simulink model "Robot_control"  (R2020b)
settings: Solver=FixedStepAuto  StartTime=0.0  StopTime=inf  FixedStep=0.01  RelTol=1e-3
values from neighbouring files (symbols this model uses):
  Initial_pos = [20 20 10]    [Robot_control_script.m]
  min_pwm_change = 0.39    [Robot_control_script.m]
  Motorspeed_MG996 = 60/.17    (= 352.941176471)    [Robot_control_script.m]
  Time_to_wait = [1 10]    [Robot_control_script.m]
  weights = [1 1 1 1 1 1]    [Robot_control_script.m]
undefined symbols (not defined in the file or in its folder): DiscIntNeverNeededParam, Levenberg, Marquardt, read_the_data, send_serial, Serial_Port, Standard_Devices
libraries: sldrtlib x4, simulink x3, robotcorelib x2, robotmaniplib x1, simulink_extras x1, dspstat3 x1, mspfiltlib x1, dspfdesign x1
(part 1 of 2)
settings Model: Creator=jsmit  LastModifiedBy=jsmit
settings OptimizationCC: DefaultParameterBehavior=Inlined  UseDivisionForNetSlopeComputation=on  GainParamInheritBuiltInType=on  UseFloatMulNetSlope=on  InlineInvariantSignals=on  EnhancedBackFolding=on  PassReuseOutputArgsAs=Individual arguments  ZeroExternalMemoryAtStartup=off  ZeroInternalMemoryAtStartup=off  EfficientFloat2IntCast=on  OptimizeBlockOrder=speed  DifferentSizesBufferReuse=on  OptimizationCustomize=off  EfficientTunableParamExpr=on
settings DebuggingCC: ParameterTunabilityLossMsg=error
settings SFSimCC: MATLABDynamicMemAllocThreshold=400000
settings RTWCC: Description=Embedded Coder  SystemTargetFile=ert.tlc  GenerateMakefile=off  TemplateMakefile=ert_default_tmf  GenerateReport=on  LaunchReport=on  TargetLang=C++  RTWCompilerOptimization=on
settings CodeAppCC: ForceParamTrailComments=on  IgnoreCustomStorageClasses=off  MaxIdLength=95  OperatorAnnotations=on  SimulinkDataObjDesc=on  SFDataObjDesc=on  InsertBlockDesc=on
settings ERTTargetCC: TargetLangStandard=C++03 (ISO)  GenerateSampleERTMain=on  CodeInterfacePackaging=C++ class  InlinedParameterPlacement=NonHierarchical  RootIOFormat=Structure reference  ERTCustomFileTemplate=example_file_process.tlc

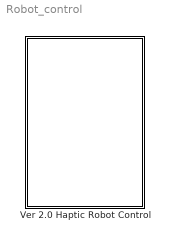
== system Robot_control ==
  Ver 2.0 Haptic Robot Control : Subsystem

== system Robot_control/Ver 2.0 Haptic Robot Control ==
  Motor Driver System : Subsystem
  Tooltip System : Subsystem  Commented=on

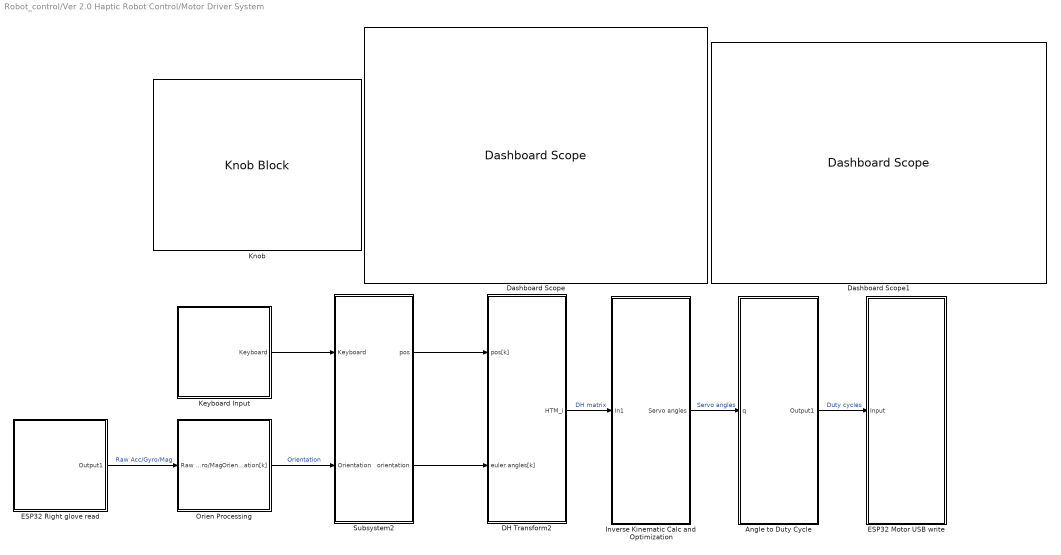
== system Robot_control/Ver 2.0 Haptic Robot Control/Motor Driver System ==
  Angle to Duty Cycle : Subsystem
  DH Transform2 : Subsystem
  Dashboard Scope : DashboardScope  TimeSpan=60  Ymin=-50  Ymax=50
  Dashboard Scope1 : DashboardScope  TimeSpan=60  Ymin=-180  Ymax=180
  ESP32 Motor USB write : Subsystem
  ESP32 Right glove read : Subsystem
  Inverse Kinematic Calc and Optimization : Subsystem
  Keyboard Input : Subsystem
  Knob : KnobBlock  ScaleMin=-40  ScaleMax=40
  Orien Processing : Subsystem
  Subsystem2 : Subsystem
  wires:
  Inverse Kinematic Calc and Optimization/1(Servo angles) -> Angle to Duty Cycle/1(q)  "Servo angles"
  Angle to Duty Cycle/1(Output1) -> ESP32 Motor USB write/1(Input)  "Duty cycles"
  ESP32 Right glove read/1(Output1) -> Orien Processing/1(Raw Acc/Gyro/Mag)  "Raw Acc/Gyro/Mag"
  DH Transform2/1(HTM_i) -> Inverse Kinematic Calc and Optimization/1(In1)  "DH matrix"
  Keyboard Input/1(Keyboard) -> Subsystem2/1(Keyboard)
  Orien Processing/1(Orientation[k]) -> Subsystem2/2(Orientation)  "Orientation"
  Subsystem2/1(pos) -> DH Transform2/1(pos[k])
  Subsystem2/2(orientation) -> DH Transform2/2(euler angles[k])

== system Robot_control/Ver 2.0 Haptic Robot Control/Tooltip System ==
  Constant : Constant  Value=100
  Counter Limited : simulink/Sources/Counter Limited  uplimit=100  tsamp=-1
  Display : Display
  ESP32 Motor USB write : Subsystem  Commented=on
  ESP32 Tooltip USB read : Subsystem
  GreaterThan : RelationalOperator  Operator===  OutDataTypeStr=boolean  RndMeth=Simplest
  Laser and Touch Processing : Subsystem  Commented=on
  Subsystem : Subsystem
  Subsystem1 : Subsystem
  wires:
  Laser and Touch Processing/1(Laser distance filtered/touch) -> ESP32 Motor USB write/1(Input)  "Tooltip Data"
  ESP32 Tooltip USB read/1(Distance/Touch) -> Subsystem1/1(Tooltip data), Laser and Touch Processing/1(Input)  "Tooltip data"
  GreaterThan/1 -> Display/1, Subsystem/Enable
  Counter Limited/1 -> GreaterThan/1
  Constant/1 -> GreaterThan/2
  Subsystem1/1(y) -> Subsystem/1(Input)

== system Robot_control/Ver 2.0 Haptic Robot Control/Motor Driver System/Angle to Duty Cycle ==
  q : Inport
  Add : Sum
  Constant : Constant  Value=0.025/60
  Constant1 : Constant  Value=0.075
  Display : Display
  Display1 : Display
  Product : Product
  Output1 : Outport
  wires:
  q/1 -> Product/2  "q"
  Constant/1 -> Product/1
  Product/1 -> Display/1, Add/2
  Constant1/1 -> Add/1
  Add/1 -> Display1/1, Output1/1  "Duty Cycle"

== system Robot_control/Ver 2.0 Haptic Robot Control/Motor Driver System/DH Transform2 ==
  pos[k] : Inport
  euler angles[k] : Inport  Port=2
  Coordinate Transformation Conversion : robotcorelib/Coordinate Transformation Conversion  InputRepresentation=Euler Angles  InputEulerSequence=XYZ  ShowTrVecInputPort=on  OutputRepresentation=Homogeneous Transformation  OutputEulerSequence=ZYX  ShowTrVecOutputPort=on  SimulateUsing=Interpreted execution
      settings: SourceProductBaseCode=NV,RO,RR,UV
  HTM_i : Outport
  wires:
  Coordinate Transformation Conversion/1 -> HTM_i/1  "i-1_A_i"
  euler angles[k]/1 -> Coordinate Transformation Conversion/1  "Euler Angles[k]"
  pos[k]/1 -> Coordinate Transformation Conversion/2  "Pos[k]"

== system Robot_control/Ver 2.0 Haptic Robot Control/Motor Driver System/ESP32 Motor USB write ==
  Input : Inport  PortDimensions=6
  Constant : Constant  Value=100
  Counter Limited : simulink/Sources/Counter Limited  uplimit=100  tsamp=-1
  Display : Display
  GreaterThan : RelationalOperator  Operator===  OutDataTypeStr=boolean  RndMeth=Simplest
  Subsystem : Subsystem
  wires:
  Constant/1 -> GreaterThan/2
  Counter Limited/1 -> GreaterThan/1
  Input/1 -> Subsystem/1(Input)  "PWM values"
  GreaterThan/1 -> Display/1, Subsystem/Enable

== system Robot_control/Ver 2.0 Haptic Robot Control/Motor Driver System/ESP32 Right glove read ==
  Triggered Subsystem : Subsystem  TreatAsAtomicUnit=on
  Output1 : Outport
  wires:
  Triggered Subsystem/1(y) -> Output1/1  "Glove Data"

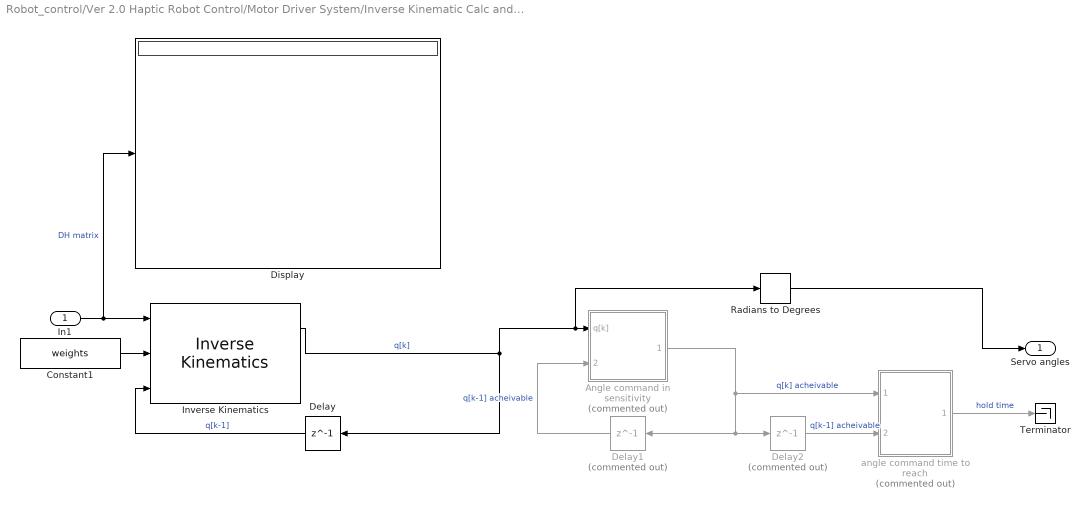
== system Robot_control/Ver 2.0 Haptic Robot Control/Motor Driver System/Inverse Kinematic Calc and Optimization ==
  In1 : Inport
  Angle command in sensitivity : Subsystem  Commented=on
  Constant1 : Constant  Value=weights
  Delay : Delay  DelayLength=1
  Delay1 : Delay  Commented=on  DelayLength=1
  Delay2 : Delay  Commented=on  DelayLength=1
  Display : Display
  Inverse Kinematics : robotmaniplib/Inverse Kinematics  RigidBodyTree=robot  EndEffector=body6  ShowInfo=off  SolverName=Levenberg-Marquardt  EnforceJointLimits=on  MaxIterations=10  MaxTime=0.3  GradientTolerance=1e-7  SolutionTolerance=0.1  StepTolerance=1e-14  ErrorChangeTolerance=0.1  UseErrorDamping=on  DampingBias=0.0025  SimulateUsing=Interpreted execution
  Radians to Degrees : simulink_extras/Transformations/Radians to Degrees
  Terminator : Terminator
  angle command time to reach : Subsystem  Commented=on
  Servo angles : Outport
  wires:
  Constant1/1 -> Inverse Kinematics/2
  Inverse Kinematics/1 -> Radians to Degrees/1, Angle command in sensitivity/1(q[k]), Delay/1  "q[k]"
  In1/1 -> Display/1, Inverse Kinematics/1  "DH matrix"
  Delay/1 -> Inverse Kinematics/3  "q[k-1]"
  Angle command in sensitivity/1(q[k] acheivable) -> Delay2/1, Delay1/1, angle command time to reach/1(q[k] acheivable)  "q[k] acheivable"
  Delay1/1 -> Angle command in sensitivity/2(q[k-1] acheivable)  "q[k-1] acheivable"
  Delay2/1 -> angle command time to reach/2(q[k-1] acheivable)  "q[k-1] acheivable"
  angle command time to reach/1(Output) -> Terminator/1  "hold time"
  Radians to Degrees/1 -> Servo angles/1

== system Robot_control/Ver 2.0 Haptic Robot Control/Motor Driver System/Keyboard Input ==
  Keyboard 1 : M-S-Function  FunctionName=sfun_keyboard_input_v1_2b  mask(Keyboard Input){}
      mask help: Keyboard Input
      mask Display: fprintf('Keyboard');
  Terminator : Terminator
  Keyboard : Outport
  wires:
  Keyboard 1/2 -> Terminator/1
  Keyboard 1/1 -> Keyboard/1

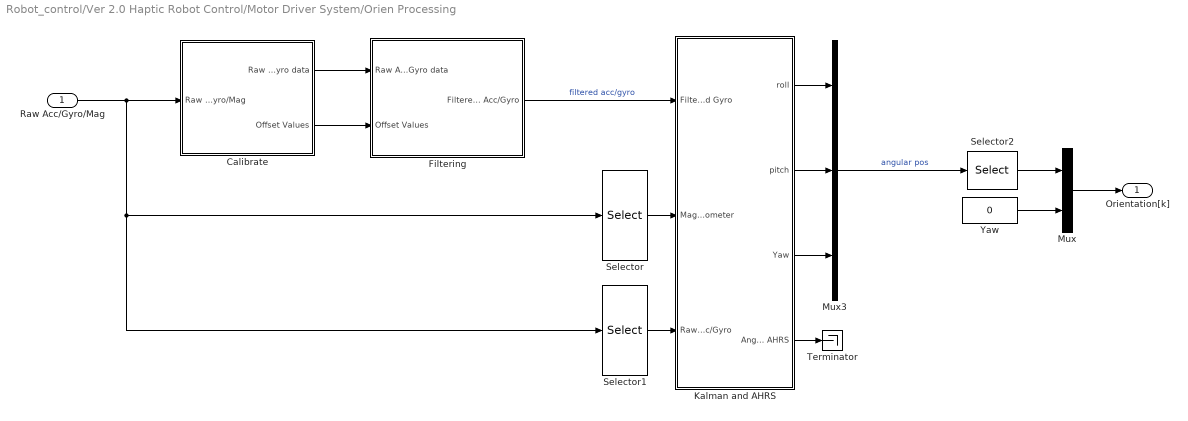
== system Robot_control/Ver 2.0 Haptic Robot Control/Motor Driver System/Orien Processing ==
  Raw Acc/Gyro/Mag : Inport
  Calibrate : Subsystem
  Filtering : Subsystem
  Kalman and AHRS : Subsystem
  Mux : Mux  Inputs=2
  Mux3 : Mux  Inputs=3
  Selector : Selector  InputPortWidth=9  IndexOptions=Index vector (dialog)  Indices=[7 8 9]  OutputSizes=1
  Selector1 : Selector  InputPortWidth=9  IndexOptions=Index vector (dialog)  Indices=[1 2 3 4 5 6]  OutputSizes=1
  Selector2 : Selector  InputPortWidth=3  IndexOptions=Index vector (dialog)  Indices=[1 2]  OutputSizes=1
  Terminator : Terminator
  Yaw : Constant  Value=0
  Orientation[k] : Outport
  wires:
  Filtering/1(Filtered Acc/Gyro) -> Kalman and AHRS/1(Filtered Acc and Gyro)  "filtered acc/gyro"
  Kalman and AHRS/3(Yaw) -> Mux3/3
  Kalman and AHRS/1(roll) -> Mux3/1
  Kalman and AHRS/2(pitch) -> Mux3/2
  Calibrate/1(Raw Acc/Gyro data) -> Filtering/1(Raw Acc/Gyro data)
  Raw Acc/Gyro/Mag/1 -> Selector1/1, Selector/1, Calibrate/1(Raw Acc/Gyro/Mag)
  Calibrate/2(Offset Values) -> Filtering/2(Offset Values)
  Mux3/1 -> Selector2/1  "angular pos"
  Selector/1 -> Kalman and AHRS/2(Magnetometer)
  Selector1/1 -> Kalman and AHRS/3(Raw Acc/Gyro)
  Selector2/1 -> Mux/1
  Mux/1 -> Orientation[k]/1
  Yaw/1 -> Mux/2
  Kalman and AHRS/4(Angular Velocity AHRS) -> Terminator/1

== system Robot_control/Ver 2.0 Haptic Robot Control/Motor Driver System/Subsystem2 ==
  Keyboard : Inport
  Orientation : Inport  Port=2
  NOT : Logic  Operator=NOT  IconShape=distinctive  AllPortsSameDT=off  OutDataTypeStr=boolean
  Saturation : Saturate  UpperLimit=40  LowerLimit=-40
  Select pos or orientation mode : Subsystem
  Subsystem : Subsystem
  pos : Outport
  orientation : Outport  Port=2
  wires:
  Select pos or orientation mode/2(pos) -> Saturation/1
  Orientation/1 -> Select pos or orientation mode/3(xy orientation), Subsystem/2(angular pos)
  NOT/1 -> Subsystem/Enable
  [A] -> Select pos or orientation mode/2(Keyboard)
  Select pos or orientation mode/3(orientation) -> orientation/1
  Select pos or orientation mode/1(In orientation mode) -> NOT/1
  Subsystem/1(xyz pos) -> Select pos or orientation mode/1(xy pos)
  [A] -> Subsystem/1(Keyboard)
  Keyboard/1 -> [A]
  Saturation/1 -> pos/1

== system Robot_control/Ver 2.0 Haptic Robot Control/Tooltip System/ESP32 Motor USB write ==
  Input : Inport  PortDimensions=6
  Constant : Constant  Value=100
  Counter Limited : simulink/Sources/Counter Limited  uplimit=100  tsamp=-1
  Display : Display
  GreaterThan : RelationalOperator  Operator===  OutDataTypeStr=boolean  RndMeth=Simplest
  Subsystem : Subsystem
  wires:
  Constant/1 -> GreaterThan/2
  Counter Limited/1 -> GreaterThan/1
  Input/1 -> Subsystem/1(Input)  "PWM values"
  GreaterThan/1 -> Display/1, Subsystem/Enable

== system Robot_control/Ver 2.0 Haptic Robot Control/Tooltip System/ESP32 Tooltip USB read ==
  Subsystem : Subsystem
  Distance/Touch : Outport
  wires:
  Subsystem/1(tool_data) -> Distance/Touch/1  "laser distance, touch"

== system Robot_control/Ver 2.0 Haptic Robot Control/Tooltip System/Laser and Touch Processing ==
  Input : Inport
  Demux : Demux  Outputs=2
  Lowpass Filter : dspfdesign/Lowpass Filter  FilterType=FIR  DesignForMinimumOrder=on  FilterOrder=50  PassbandFrequency=8e3  StopbandFrequency=12e3  PassbandRipple=0.1  StopbandAttenuation=80  InheritSampleRate=off  SampleRate=44100  SimulateUsing=Interpreted execution  roundingMode=Floor  coeffsDataTypeStr=fixdt(1,16)
  Mux : Mux  Inputs=2
  Subsystem : Subsystem
  Laser distance filtered/touch : Outport
  wires:
  Input/1 -> Demux/1  "Tooltip data[k]"
  Demux/1 -> Lowpass Filter/1  "Laser distance[k]"
  Lowpass Filter/1 -> Mux/1
  Mux/1 -> Laser distance filtered/touch/1
  Demux/2 -> Subsystem/1(Tiptouch[k])  "Tiptouch[k]"
  Subsystem/1(Tool touching last 3 samples) -> Mux/2

== system Robot_control/Ver 2.0 Haptic Robot Control/Tooltip System/Subsystem ==
  Input : Inport  PortDimensions=[1 2]
  Enable : EnablePort
  Display : Display
  Display1 : Display
  Interpreted MATLAB Function : MATLABFcn  MATLABFcn=send_serial(u)  OutputDimensions=0
  Stream Output1 : sldrtlib/Stream Output  Commented=on  SampleTime=0.01  MaxMissedTicks=inf  ShowMissedTicks=off  YieldWhenWaiting=off  DrvName=Standard_Devices/Serial_Port  DrvAddress=4  DrvOptions=[115200 8 0 0 0 0 0 0]  PortSizes=1  FormatString='%s'  ShowReady=off  ShowError=off  InitialValue=[]  FinalValue=[]
      settings: AttributesFormatString=Serial Port [4]  SourceProductBaseCode=WT
  wires:
  Input/1 -> Display1/1, Interpreted MATLAB Function/1

== system Robot_control/Ver 2.0 Haptic Robot Control/Tooltip System/Subsystem1 ==
  Tooltip data : Inport
  Display : Display
  Display1 : Display
  MATLAB Function1 : MATLAB Function  TreatAsAtomicUnit=on
  y : Outport  PortDimensions=[1 2]
  wires:
  Tooltip data/1 -> Display/1, MATLAB Function1/1(my_string)
  MATLAB Function1/1(y) -> Display1/1, y/1

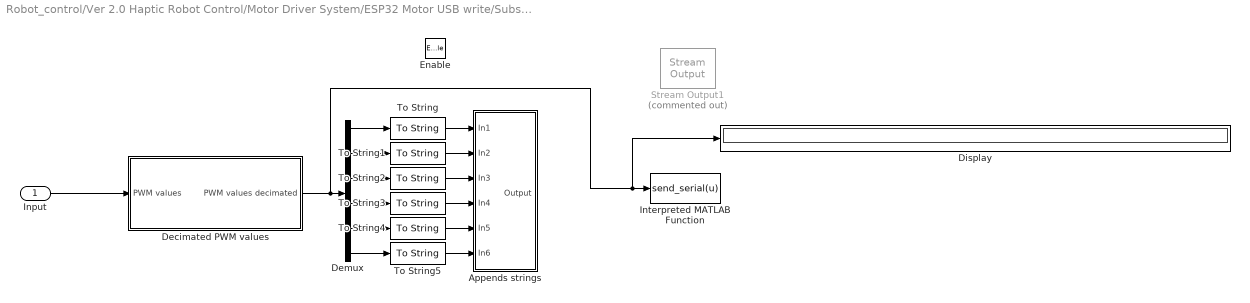
== system Robot_control/Ver 2.0 Haptic Robot Control/Motor Driver System/ESP32 Motor USB write/Subsystem ==
  Input : Inport  PortDimensions=6
  Enable : EnablePort
  Appends strings : Subsystem
  Decimated PWM values : Subsystem
  Demux : Demux  Outputs=6
  Display : Display
  Interpreted MATLAB Function : MATLABFcn  MATLABFcn=send_serial(u)  OutputDimensions=0
  Stream Output1 : sldrtlib/Stream Output  Commented=on  SampleTime=0.01  MaxMissedTicks=inf  ShowMissedTicks=off  YieldWhenWaiting=off  DrvName=Standard_Devices/Serial_Port  DrvAddress=4  DrvOptions=[115200 8 0 0 0 0 0 0]  PortSizes=1  FormatString='%s'  ShowReady=off  ShowError=off  InitialValue=[]  FinalValue=[]
      settings: AttributesFormatString=Serial Port [4]  SourceProductBaseCode=WT
  To String{,1..5} (6 alike) : ToString
  wires:
  Demux/3 -> To String2/1
  To String4/1 -> Appends strings/5(In5)
  Demux/6 -> To String5/1
  To String3/1 -> Appends strings/4(In4)
  Demux/1 -> To String/1
  To String2/1 -> Appends strings/3(In3)
  To String5/1 -> Appends strings/6(In6)
  To String1/1 -> Appends strings/2(In2)
  To String/1 -> Appends strings/1(In1)
  Demux/4 -> To String3/1
  Decimated PWM values/1(PWM values decimated) -> Display/1, Interpreted MATLAB Function/1, Demux/1
  Demux/2 -> To String1/1
  Demux/5 -> To String4/1
  Input/1 -> Decimated PWM values/1(PWM values)

== system Robot_control/Ver 2.0 Haptic Robot Control/Motor Driver System/ESP32 Right glove read/Triggered Subsystem ==
  Gain : Gain  Gain=1/100
  Interpreted MATLAB Function : MATLABFcn  Commented=on  MATLABFcn=read_the_data(u)
  MATLAB Function1 : MATLAB Function  TreatAsAtomicUnit=on
  Stream Input : sldrtlib/Stream Input  SampleTime=0.01  MaxMissedTicks=inf  ShowMissedTicks=off  YieldWhenWaiting=off  DrvName=Standard_Devices/Serial_Port  DrvAddress=8  DrvOptions=[9600 8 0 0 0 0 0 0]  DataTypes='string'  FormatString='%s'  Terminator={'\r', '\n'}  ShowReady=off  ShowError=off
      settings: AttributesFormatString=Serial Port [8]  SourceProductBaseCode=WT
  y : Outport  OutDataTypeStr=double
  wires:
  Stream Input/1 -> Interpreted MATLAB Function/1, MATLAB Function1/1(my_string)
  Gain/1 -> y/1
  MATLAB Function1/1(y) -> Gain/1

== system Robot_control/Ver 2.0 Haptic Robot Control/Motor Driver System/Inverse Kinematic Calc and Optimization/Angle command in sensitivity ==
  q[k] : Inport
  q[k-1] acheivable : Inport  Port=2
  Angle to duty cycle : Subsystem
  Subtract : Sum  Inputs=+-
  q[k] acheivable : Outport
  wires:
  q[k]/1 -> Angle to duty cycle/1(q[k]), Subtract/1  "q[k]"
  q[k-1] acheivable/1 -> Subtract/2, Angle to duty cycle/3(Input1)  "q[k-1] acheivable"
  Angle to duty cycle/1(q[k] acheiveable) -> q[k] acheivable/1
  Subtract/1 -> Angle to duty cycle/2(Angle change)  "angle change"

== system Robot_control/Ver 2.0 Haptic Robot Control/Motor Driver System/Inverse Kinematic Calc and Optimization/angle command time to reach ==
  q[k] acheivable : Inport
  q[k-1] acheivable : Inport  Port=2
  Constant1 : Constant  Value=Motorspeed_MG996
  Divide : Product  Inputs=/*
  Max : MinMax  Function=max
  Subtract : Sum  Inputs=+-
  Output : Outport
  wires:
  Constant1/1 -> Divide/1
  Max/1 -> Divide/2
  Divide/1 -> Output/1
  q[k-1] acheivable/1 -> Subtract/2
  q[k] acheivable/1 -> Subtract/1
  Subtract/1 -> Max/1

== system Robot_control/Ver 2.0 Haptic Robot Control/Motor Driver System/Orien Processing/Calibrate ==
  Raw Acc/Gyro/Mag : Inport
  Calculate offset values : Subsystem
  Pass 0's until Offset Calc. : Subsystem
  Selector : Selector  InputPortWidth=9  IndexOptions=Index vector (dialog)  Indices=[1 2 3 4 5 6]  OutputSizes=1
  Raw Acc/Gyro data : Outport
  Offset Values : Outport  Port=2
  wires:
  Raw Acc/Gyro/Mag/1 -> Selector/1
  Selector/1 -> Calculate offset values/1(Acc and Ang vel), Pass 0's until Offset Calc./1(In1)
  Pass 0's until Offset Calc./1(Out1) -> Raw Acc/Gyro data/1
  Calculate offset values/1(Offset Values) -> Offset Values/1

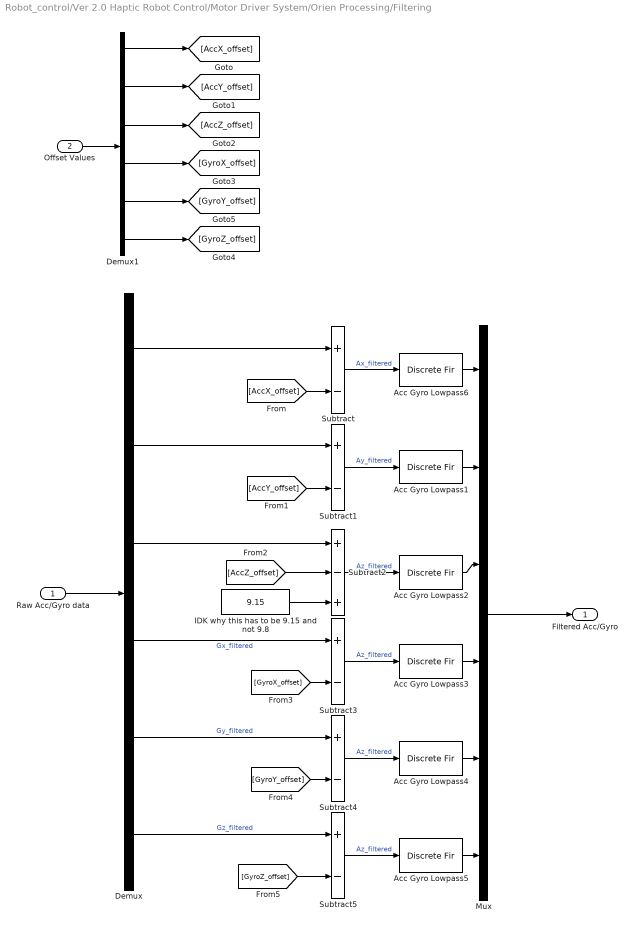
== system Robot_control/Ver 2.0 Haptic Robot Control/Motor Driver System/Orien Processing/Filtering ==
  Raw Acc/Gyro data : Inport
  Offset Values : Inport  Port=2
  Acc Gyro Lowpass{1..6} (6 alike) : DiscreteFir  Tag=BlockMethodSubSystem  Coefficients=[-0.00268886099103231432 -0.00550842062906714645 0.0207886441632320826 0.114078459669350679 0.246264331684130783 0.311632819991308929 0.246264331684130783 0.114078459669350679 0.0207886441632320826 -0.00550842062906714645 -0.00268886099103231432]  InputProcessing=Columns as channels (frame based)
  Demux : Demux  Outputs=6
  Demux1 : Demux  Outputs=6
  IDK why this has to be 9.15 and not 9.8 : Constant  Value=9.15
  Mux : Mux  Inputs=6
  Subtract{,1,3..5} (5 alike) : Sum  Inputs=+-
  Subtract2 : Sum  Inputs=+-+
  Filtered Acc/Gyro : Outport
  wires:
  [AccX_offset] -> Subtract/2
  Subtract/1 -> Acc Gyro Lowpass6/1  "Ax_filtered"
  Subtract2/1 -> Acc Gyro Lowpass2/1  "Az_filtered"
  [AccY_offset] -> Subtract1/2
  Subtract1/1 -> Acc Gyro Lowpass1/1  "Ay_filtered"
  Demux1/1 -> [AccX_offset]
  Demux1/2 -> [AccY_offset]
  Demux1/3 -> [AccZ_offset]
  Demux1/4 -> [GyroX_offset]
  Demux1/5 -> [GyroY_offset]
  Demux1/6 -> [GyroZ_offset]
  Offset Values/1 -> Demux1/1
  Demux/6 -> Subtract5/1  "Gz_filtered"
  Demux/5 -> Subtract4/1  "Gy_filtered"
  Demux/4 -> Subtract3/1  "Gx_filtered"
  Subtract3/1 -> Acc Gyro Lowpass3/1  "Az_filtered"
  Subtract4/1 -> Acc Gyro Lowpass4/1  "Az_filtered"
  Subtract5/1 -> Acc Gyro Lowpass5/1  "Az_filtered"
  Raw Acc/Gyro data/1 -> Demux/1
  [GyroX_offset] -> Subtract3/2
  [GyroY_offset] -> Subtract4/2
  Demux/1 -> Subtract/1
  Demux/2 -> Subtract1/1
  Demux/3 -> Subtract2/1
  [GyroZ_offset] -> Subtract5/2
  [AccZ_offset] -> Subtract2/2
  Acc Gyro Lowpass6/1 -> Mux/1
  Acc Gyro Lowpass1/1 -> Mux/2
  Acc Gyro Lowpass2/1 -> Mux/3
  Acc Gyro Lowpass3/1 -> Mux/4
  Acc Gyro Lowpass4/1 -> Mux/5
  Acc Gyro Lowpass5/1 -> Mux/6
  IDK why this has to be 9.15 and not 9.8/1 -> Subtract2/3
  Mux/1 -> Filtered Acc/Gyro/1

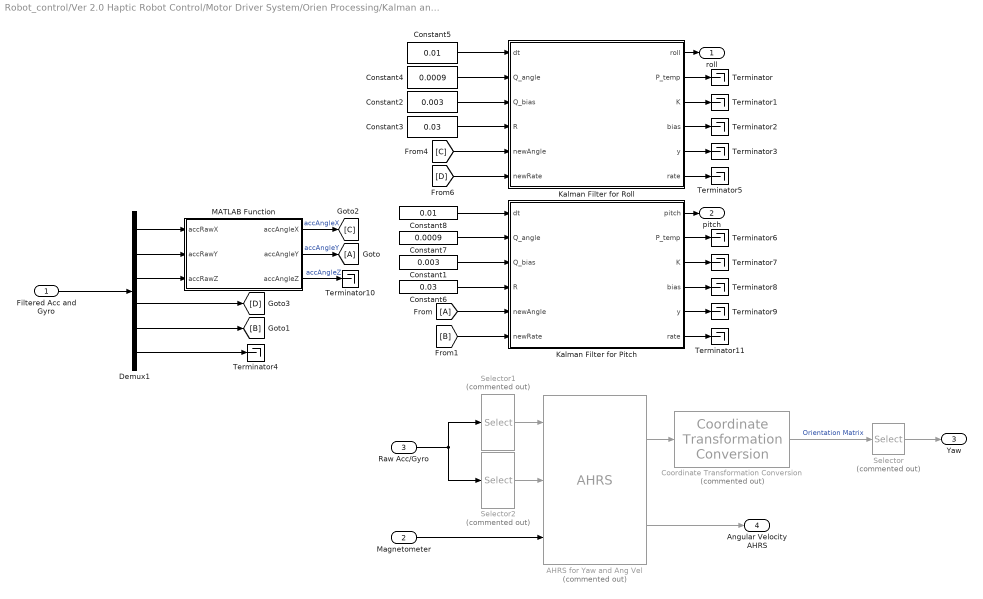
== system Robot_control/Ver 2.0 Haptic Robot Control/Motor Driver System/Orien Processing/Kalman and AHRS ==
  Filtered Acc and Gyro : Inport
  Magnetometer : Inport  Port=2
  Raw Acc/Gyro : Inport  Port=3
  AHRS for Yaw and Ang Vel : mspfiltlib/AHRS  Commented=on  DispRefFrame=NED  DecimationFactor=1  InitialProcessNoise=ahrsfilter.defaultProcessNoise  OrientationFormat=Rotation matrix  SimulateUsing=Interpreted execution  AccelerometerNoise=0.0001924722  GyroscopeNoise=9.1385e-5  MagnetometerNoise=0.1  GyroscopeDriftNoise=3.0462e-13  LinearAccelerationNoise=0.0096236100000000012  MagneticDisturbanceNoise=0.5  LinearAccelerationDecayFactor=0.5  MagneticDisturbanceDecayFactor=0.5  ExpectedMagneticFieldStrength=50
      settings: SourceProductBaseCode=TF,NV
  Constant1 : Constant  Value=0.003
  Constant2 : Constant  Value=0.003
  Constant3 : Constant  Value=0.03
  Constant4 : Constant  Value=0.0009
  Constant5 : Constant  Value=0.01
  Constant6 : Constant  Value=0.03
  Constant7 : Constant  Value=0.0009
  Constant8 : Constant  Value=0.01
  Coordinate Transformation Conversion : robotcorelib/Coordinate Transformation Conversion  Commented=on  InputRepresentation=Rotation Matrix  InputEulerSequence=XYZ  ShowTrVecInputPort=off  OutputRepresentation=Euler Angles  OutputEulerSequence=XYZ  ShowTrVecOutputPort=on  SimulateUsing=Interpreted execution
      settings: SourceProductBaseCode=NV,RO,RR,UV
  Demux1 : Demux  Outputs=6
  Kalman Filter for Pitch : MATLAB Function  TreatAsAtomicUnit=on
  Kalman Filter for Roll : MATLAB Function  TreatAsAtomicUnit=on
  MATLAB Function : MATLAB Function  TreatAsAtomicUnit=on
  Selector : Selector  Commented=on  InputPortWidth=3  IndexOptions=Index vector (dialog)  Indices=[3]  OutputSizes=1
  Selector1 : Selector  Commented=on  InputPortWidth=6  IndexOptions=Index vector (dialog)  Indices=[1 2 3]  OutputSizes=1
  Selector2 : Selector  Commented=on  InputPortWidth=6  IndexOptions=Index vector (dialog)  Indices=[4 5 6]  OutputSizes=1
  Terminator{,1..11} (12 alike) : Terminator
  roll : Outport
  pitch : Outport  Port=2
  Yaw : Outport  Port=3
  Angular Velocity AHRS : Outport  Port=4
  wires:
  Constant3/1 -> Kalman Filter for Roll/4(R)
  [A] -> Kalman Filter for Pitch/5(newAngle)
  Demux1/3 -> MATLAB Function/3(accRawZ)
  Kalman Filter for Roll/5(y) -> Terminator3/1
  Constant7/1 -> Kalman Filter for Pitch/2(Q_angle)
  MATLAB Function/1(accAngleX) -> [C]  "accAngleX"
  Kalman Filter for Pitch/4(bias) -> Terminator8/1
  [C] -> Kalman Filter for Roll/5(newAngle)
  Kalman Filter for Roll/1(roll) -> roll/1
  Constant2/1 -> Kalman Filter for Roll/3(Q_bias)
  Kalman Filter for Roll/6(rate) -> Terminator5/1
  [D] -> Kalman Filter for Roll/6(newRate)
  Demux1/6 -> Terminator4/1
  Constant8/1 -> Kalman Filter for Pitch/1(dt)
  Demux1/5 -> [B]
  Kalman Filter for Roll/2(P_temp) -> Terminator/1
  Kalman Filter for Pitch/3(K) -> Terminator7/1
  Constant6/1 -> Kalman Filter for Pitch/4(R)
  Demux1/2 -> MATLAB Function/2(accRawY)
  Filtered Acc and Gyro/1 -> Demux1/1
  Demux1/1 -> MATLAB Function/1(accRawX)
  Demux1/4 -> [D]
  Constant5/1 -> Kalman Filter for Roll/1(dt)
  Constant4/1 -> Kalman Filter for Roll/2(Q_angle)
  Kalman Filter for Roll/3(K) -> Terminator1/1
  Kalman Filter for Pitch/2(P_temp) -> Terminator6/1
  Kalman Filter for Pitch/6(rate) -> Terminator11/1
  MATLAB Function/2(accAngleY) -> [A]  "accAngleY"
  Kalman Filter for Roll/4(bias) -> Terminator2/1
  Kalman Filter for Pitch/5(y) -> Terminator9/1
  [B] -> Kalman Filter for Pitch/6(newRate)
  Constant1/1 -> Kalman Filter for Pitch/3(Q_bias)
  Kalman Filter for Pitch/1(pitch) -> pitch/1
  MATLAB Function/3(accAngleZ) -> Terminator10/1  "accAngleZ"
  Selector/1 -> Yaw/1
  Magnetometer/1 -> AHRS for Yaw and Ang Vel/3
  Raw Acc/Gyro/1 -> Selector2/1, Selector1/1
  Selector1/1 -> AHRS for Yaw and Ang Vel/1
  Selector2/1 -> AHRS for Yaw and Ang Vel/2
  AHRS for Yaw and Ang Vel/2 -> Angular Velocity AHRS/1
  AHRS for Yaw and Ang Vel/1 -> Coordinate Transformation Conversion/1
  Coordinate Transformation Conversion/1 -> Selector/1  "Orientation Matrix"

== system Robot_control/Ver 2.0 Haptic Robot Control/Motor Driver System/Subsystem2/Select pos or orientation mode ==
  note: p=position=112
  note: o=orientation 111
  xy pos : Inport
  Keyboard : Inport  Port=2
  xy orientation : Inport  Port=3
  If keyboard changes from o->p or p->o then wait 3 sec : Subsystem
  Use glove for Pos : Subsystem
  use glove for Orien : Subsystem
  In orientation mode : Outport
  pos : Outport  Port=2
  orientation : Outport  Port=3
  wires:
  Keyboard/1 -> use glove for Orien/2(In2), Use glove for Pos/1(In1), If keyboard changes from o->p or p->o then wait 3 sec/1(In1)
  xy orientation/1 -> use glove for Orien/1(In1)
  use glove for Orien/1(Out1) -> orientation/1
  xy pos/1 -> Use glove for Pos/2(In2)
  Use glove for Pos/1(Out1) -> pos/1
  use glove for Orien/2(In orientation mode) -> In orientation mode/1

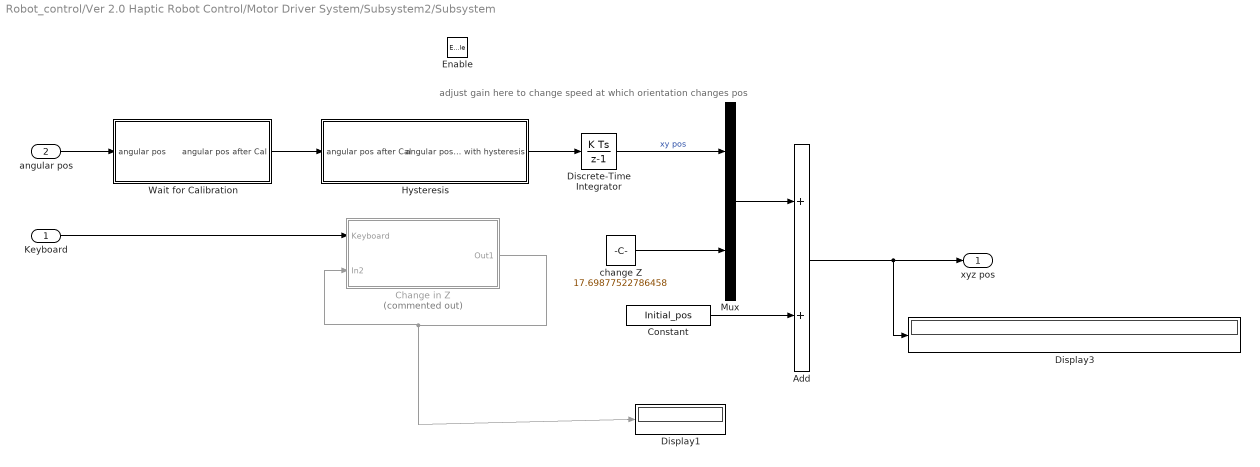
== system Robot_control/Ver 2.0 Haptic Robot Control/Motor Driver System/Subsystem2/Subsystem ==
  note: adjust gain here to change speed at which orientation changes pos
  Keyboard : Inport
  angular pos : Inport  Port=2
  Enable : EnablePort
  Add : Sum
  Change in Z : Subsystem  Commented=on
  Constant : Constant  Value=Initial_pos
  Discrete-Time Integrator : DiscreteIntegrator  gainval=1/10  SampleTime=-1  ICPrevOutput=DiscIntNeverNeededParam  ICPrevScaledInput=DiscIntNeverNeededParam
  Display1 : Display
  Display3 : Display
  Hysteresis : Subsystem
  Mux : Mux  Inputs=2
  Wait for Calibration : Subsystem
  change Z : Constant  Value=17.69877522786458
  xyz pos : Outport
  wires:
  angular pos/1 -> Wait for Calibration/1(angular pos)
  Wait for Calibration/1(angular pos after Cal) -> Hysteresis/1(angular pos after Cal)
  Hysteresis/1(angular pos with hysteresis) -> Discrete-Time Integrator/1
  Add/1 -> xyz pos/1, Display3/1
  Discrete-Time Integrator/1 -> Mux/1  "xy pos"
  Mux/1 -> Add/1
  Constant/1 -> Add/2
  Change in Z/1(Out1) -> Change in Z/2(In2), Display1/1
  Keyboard/1 -> Change in Z/1(Keyboard)
  change Z/1 -> Mux/2

== system Robot_control/Ver 2.0 Haptic Robot Control/Tooltip System/ESP32 Motor USB write/Subsystem ==
  Input : Inport  PortDimensions=6
  Enable : EnablePort
  Decimated PWM values : Subsystem
  Interpreted MATLAB Function : MATLABFcn  MATLABFcn=send_serial(u)  OutputDimensions=0
  wires:
  Input/1 -> Decimated PWM values/1(PWM values)
  Decimated PWM values/1(PWM values decimated) -> Interpreted MATLAB Function/1

== system Robot_control/Ver 2.0 Haptic Robot Control/Tooltip System/ESP32 Tooltip USB read/Subsystem ==
  Display : Display
  Stream Input : sldrtlib/Stream Input  SampleTime=0.01  MaxMissedTicks=inf  ShowMissedTicks=off  YieldWhenWaiting=off  DrvName=Standard_Devices/Serial_Port  DrvAddress=6  DrvOptions=[115200 8 0 0 0 0 0 0]  DataTypes='string'  FormatString='%s'  Terminator={'\r', '\n'}  ShowReady=off  ShowError=off
      settings: AttributesFormatString=Serial Port [6]  SourceProductBaseCode=WT
  tool_data : Outport
  wires:
  Stream Input/1 -> Display/1, tool_data/1

== system Robot_control/Ver 2.0 Haptic Robot Control/Tooltip System/Laser and Touch Processing/Subsystem ==
  Tiptouch[k] : Inport
  Add : Sum  Inputs=+++
  Constant : Constant
  Constant1 : Constant  Value=0
  Delay : Delay
  Delay1 : Delay  DelayLength=1
  Switch : Switch  Threshold=3
  Tool touching last 3 samples : Outport
  wires:
  Constant1/1 -> Switch/3
  Tiptouch[k]/1 -> Delay/1, Add/1, Delay1/1
  Constant/1 -> Switch/1
  Delay/1 -> Add/3
  Add/1 -> Switch/2
  Switch/1 -> Tool touching last 3 samples/1  "Tool touching last 3 samples"
  Delay1/1 -> Add/2

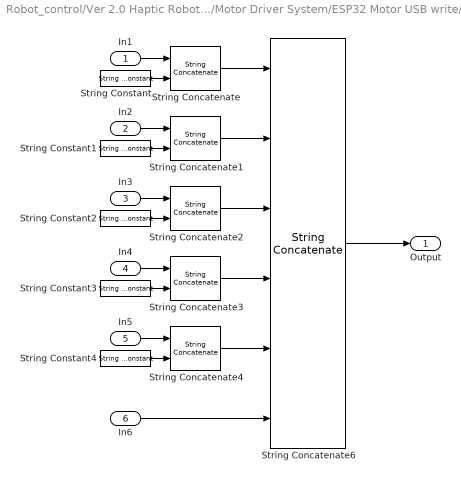
== system Robot_control/Ver 2.0 Haptic Robot Control/Motor Driver System/ESP32 Motor USB write/Subsystem/Appends strings ==
  In1 : Inport
  In2 : Inport  Port=2
  In3 : Inport  Port=3
  In4 : Inport  Port=4
  In5 : Inport  Port=5
  In6 : Inport  Port=6
  String Concatenate{,1..4} (5 alike) : StringConcatenate
  String Concatenate6 : StringConcatenate  Inputs=6
  String Constant{,1..4} (5 alike) : StringConstant  String="\" \""
  Output : Outport
  wires:
  String Concatenate/1 -> String Concatenate6/1
  String Constant/1 -> String Concatenate/2
  In1/1 -> String Concatenate/1
  String Concatenate1/1 -> String Concatenate6/2
  In2/1 -> String Concatenate1/1
  String Constant1/1 -> String Concatenate1/2
  String Concatenate2/1 -> String Concatenate6/3
  In3/1 -> String Concatenate2/1
  String Constant2/1 -> String Concatenate2/2
  In5/1 -> String Concatenate4/1
  String Concatenate3/1 -> String Concatenate6/4
  String Constant3/1 -> String Concatenate3/2
  In6/1 -> String Concatenate6/6
  In4/1 -> String Concatenate3/1
  String Constant4/1 -> String Concatenate4/2
  String Concatenate4/1 -> String Concatenate6/5
  String Concatenate6/1 -> Output/1

== system Robot_control/Ver 2.0 Haptic Robot Control/Motor Driver System/ESP32 Motor USB write/Subsystem/Decimated PWM values ==
  PWM values : Inport
  Gain : Gain  Gain=1000
  Gain1 : Gain  Gain=1/1000
  Round : Rounding
  PWM values decimated : Outport
  wires:
  Gain/1 -> Round/1
  Gain1/1 -> PWM values decimated/1
  Round/1 -> Gain1/1
  PWM values/1 -> Gain/1

== system Robot_control/Ver 2.0 Haptic Robot Control/Motor Driver System/Inverse Kinematic Calc and Optimization/Angle command in sensitivity/Angle to duty cycle ==
  q[k] : Inport
  Angle change : Inport  Port=2
  Input1 : Inport  Port=3
  Gain : Gain  Gain=1/24
  Motor move selection : Subsystem
  Mux : Mux  Inputs=3
  q[k] acheiveable : Outport
  wires:
  q[k]/1 -> Mux/1  "q[k]"
  Motor move selection/1(q[k] acheivable) -> q[k] acheiveable/1
  Input1/1 -> Mux/3  "q[k-1] ach"
  Mux/1 -> Motor move selection/1("q[k],pwm change, q[k-1] ach")
  Gain/1 -> Mux/2  "Pwm change"
  Angle change/1 -> Gain/1  "Angle change"

== system Robot_control/Ver 2.0 Haptic Robot Control/Motor Driver System/Orien Processing/Calibrate/Calculate offset values ==
  Acc and Ang vel : Inport
  Delay : Delay  DelayLength=1
  In time window to calibrate : Subsystem
  Mean : dspstat3/Mean  run=on  InputProcessing=Columns as channels (frame based)  reset_popup=None  directionMode=Each column  dimension=[1 6]  roiEnable=off  roiType=Rectangles  roiPortion=Entire ROI  roiOutput=Individual statistics for each ROI  roiFlag=off  roundingMode=Floor  overflowMode=off  outputDataTypeStr=Inherit: Same as accumulator  outputMin=[]  outputMax=[]  outputLastDataTypeStr=Inherit: Same as accumulator
  Switch1 : Switch  Criteria=u2 ~= 0  Threshold=Time_to_wait
  Offset Values : Outport
  wires:
  Switch1/1 -> Mean/1
  Mean/1 -> Offset Values/1, Delay/1  "Offset Values"
  Acc and Ang vel/1 -> Switch1/1
  In time window to calibrate/1(Out1) -> Switch1/2  "1 if in Calibrate mode, 0 else"
  Delay/1 -> Switch1/3

== system Robot_control/Ver 2.0 Haptic Robot Control/Motor Driver System/Orien Processing/Calibrate/Pass 0's until Offset Calc. ==
  In1 : Inport
  Clock : Clock
  Constant1 : Constant  Value=[0 0 0 0 0 0]
  Switch : Switch  Threshold=Time_to_wait(2)
  Out1 : Outport
  wires:
  Clock/1 -> Switch/2
  In1/1 -> Switch/1
  Constant1/1 -> Switch/3
  Switch/1 -> Out1/1

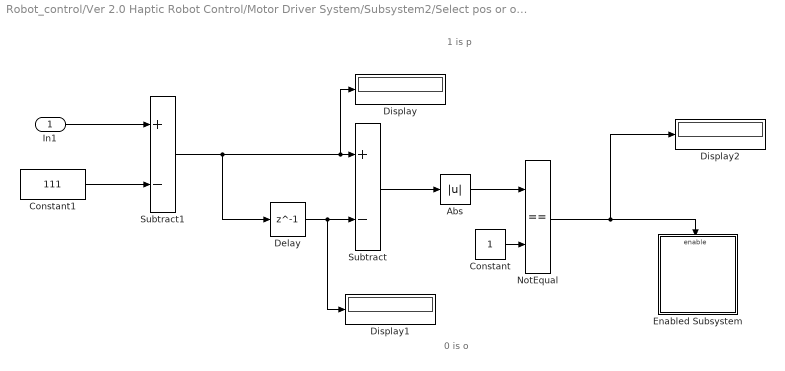
== system Robot_control/Ver 2.0 Haptic Robot Control/Motor Driver System/Subsystem2/Select pos or orientation mode/If keyboard changes from o->p or p->o then wait 3 sec ==
  note: 0 is o
  note: 1 is p
  In1 : Inport
  Abs : Abs
  Constant : Constant
  Constant1 : Constant  Value=111
  Delay : Delay  DelayLength=1
  Display : Display
  Display1 : Display
  Display2 : Display
  Enabled Subsystem : Subsystem  TreatAsAtomicUnit=on
  NotEqual : RelationalOperator  Operator===  OutDataTypeStr=boolean  RndMeth=Simplest
  Subtract : Sum  Inputs=+-
  Subtract1 : Sum  Inputs=+-
  wires:
  Delay/1 -> Display1/1, Subtract/2
  Subtract/1 -> Abs/1
  Constant/1 -> NotEqual/2
  NotEqual/1 -> Display2/1, Enabled Subsystem/Enable
  Abs/1 -> NotEqual/1
  In1/1 -> Subtract1/1
  Subtract1/1 -> Delay/1, Display/1, Subtract/1
  Constant1/1 -> Subtract1/2

== system Robot_control/Ver 2.0 Haptic Robot Control/Motor Driver System/Subsystem2/Select pos or orientation mode/Use glove for Pos ==
  In1 : Inport
  In2 : Inport  Port=2
  Constant : Constant  Value=112
  Equal : RelationalOperator  Operator===  OutDataTypeStr=boolean  RndMeth=Simplest
  Switch2 : Switch  Criteria=u2 ~= 0
  Out1 : Outport
  wires:
  Switch2/1 -> Switch2/3, Out1/1
  In2/1 -> Switch2/1
  Constant/1 -> Equal/2
  In1/1 -> Equal/1
  Equal/1 -> Switch2/2

== system Robot_control/Ver 2.0 Haptic Robot Control/Motor Driver System/Subsystem2/Select pos or orientation mode/use glove for Orien ==
  In1 : Inport
  In2 : Inport  Port=2
  Constant : Constant  Value=111
  Display : Display
  Display1 : Display
  Display2 : Display
  Equal : RelationalOperator  Operator===  OutDataTypeStr=boolean  RndMeth=Simplest
  Switch : Switch  Criteria=u2 ~= 0
  Out1 : Outport
  In orientation mode : Outport  Port=2
  wires:
  Switch/1 -> Switch/3, Display1/1, Out1/1
  In1/1 -> Display/1, Switch/1
  In2/1 -> Equal/1
  Equal/1 -> Display2/1, In orientation mode/1, Switch/2
  Constant/1 -> Equal/2

== system Robot_control/Ver 2.0 Haptic Robot Control/Motor Driver System/Subsystem2/Subsystem/Change in Z ==
  Keyboard : Inport
  In2 : Inport  Port=2
  Add2 : Sum
  Constant1 : Constant  Value=0
  Delay1 : Delay  DelayLength=1  InitialCondition=0  SampleTime=0.5
  Gain : Gain  Gain=0.2
  Switch : Switch  Criteria=u2 ~= 0
  w up 1cm s down 1cm : Subsystem
  Out1 : Outport
  wires:
  Add2/1 -> Out1/1
  Switch/1 -> Add2/1
  w up 1cm s down 1cm/1(Out1) -> Switch/2, Gain/1
  Delay1/1 -> Add2/2
  Constant1/1 -> Switch/3
  In2/1 -> Delay1/1
  Keyboard/1 -> w up 1cm s down 1cm/1(Keyboard)
  Gain/1 -> Switch/1

== system Robot_control/Ver 2.0 Haptic Robot Control/Motor Driver System/Subsystem2/Subsystem/Hysteresis ==
  angular pos after Cal : Inport
  Constant : Constant  Value=[0 0]
  Relay : Relay  OnSwitchValue=7  OffSwitchValue=4
  Selector : Selector  InputPortWidth=3  IndexOptions=Index vector (dialog)  Indices=[1 2]  OutputSizes=1
  Subsystem : Subsystem
  Switch : Switch  Criteria=u2 ~= 0
  angular pos with hysteresis : Outport
  wires:
  angular pos after Cal/1 -> Selector/1
  Constant/1 -> Switch/3
  Relay/1 -> Switch/2
  Switch/1 -> angular pos with hysteresis/1
  Subsystem/1(angular pos magnitude) -> Relay/1
  Selector/1 -> Switch/1, Subsystem/1(angular pos after Cal)

== system Robot_control/Ver 2.0 Haptic Robot Control/Motor Driver System/Subsystem2/Subsystem/Wait for Calibration ==
  angular pos : Inport
  Clock : Clock
  Constant1 : Constant  Value=Time_to_wait(2) + 1
  Constant2 : Constant  Value=[0 0 0]
  GreaterThan : RelationalOperator  Operator=>  OutDataTypeStr=boolean  RndMeth=Simplest
  Switch1 : Switch  Criteria=u2 ~= 0
  angular pos after Cal : Outport
  wires:
  Constant1/1 -> GreaterThan/2
  GreaterThan/1 -> Switch1/2
  Constant2/1 -> Switch1/3
  angular pos/1 -> Switch1/1
  Clock/1 -> GreaterThan/1
  Switch1/1 -> angular pos after Cal/1

== system Robot_control/Ver 2.0 Haptic Robot Control/Tooltip System/ESP32 Motor USB write/Subsystem/Decimated PWM values ==
  PWM values : Inport
  Gain : Gain  Gain=1000
  Gain1 : Gain  Gain=1/1000
  Round : Rounding
  PWM values decimated : Outport
  wires:
  Gain/1 -> Round/1
  Gain1/1 -> PWM values decimated/1
  Round/1 -> Gain1/1
  PWM values/1 -> Gain/1

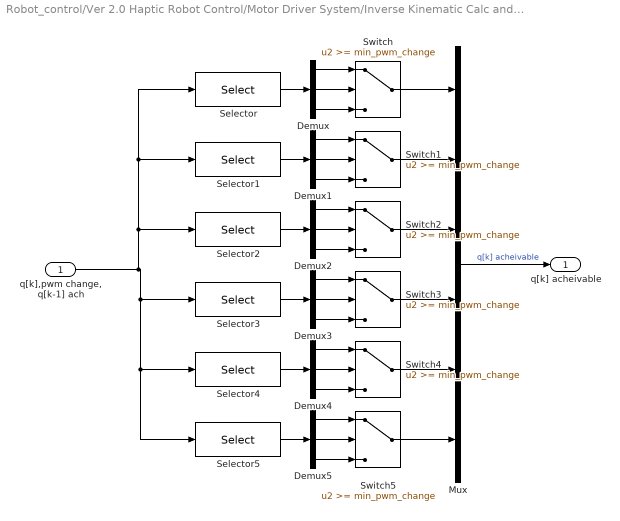
== system Robot_control/Ver 2.0 Haptic Robot Control/Motor Driver System/Inverse Kinematic Calc and Optimization/Angle command in sensitivity/Angle to duty cycle/Motor move selection ==
  "q[k],pwm change, q[k-1] ach" : Inport
  Demux{,1..5} (6 alike) : Demux  Outputs=3
  Mux : Mux  Inputs=6
  Selector : Selector  InputPortWidth=18  IndexOptions=Index vector (dialog)  Indices=[1 7 13]  OutputSizes=1
  Selector1 : Selector  InputPortWidth=18  IndexOptions=Index vector (dialog)  Indices=[2 8 14]  OutputSizes=1
  Selector2 : Selector  InputPortWidth=18  IndexOptions=Index vector (dialog)  Indices=[3 9 15]  OutputSizes=1
  Selector3 : Selector  InputPortWidth=18  IndexOptions=Index vector (dialog)  Indices=[4 10 16]  OutputSizes=1
  Selector4 : Selector  InputPortWidth=18  IndexOptions=Index vector (dialog)  Indices=[5 11 17]  OutputSizes=1
  Selector5 : Selector  InputPortWidth=18  IndexOptions=Index vector (dialog)  Indices=[6 12 18]  OutputSizes=1
  Switch{,1..5} (6 alike) : Switch  Threshold=min_pwm_change
  q[k] acheivable : Outport
  wires:
  Mux/1 -> q[k] acheivable/1  "q[k] acheivable"
  Switch5/1 -> Mux/6
  Switch4/1 -> Mux/5
  Switch3/1 -> Mux/4
  Switch2/1 -> Mux/3
  Switch1/1 -> Mux/2
  Switch/1 -> Mux/1
  Demux/1 -> Switch/1
  Demux/2 -> Switch/2
  Demux/3 -> Switch/3
  Demux1/1 -> Switch1/1
  Demux1/2 -> Switch1/2
  Demux1/3 -> Switch1/3
  Demux2/1 -> Switch2/1
  Demux2/2 -> Switch2/2
  Demux2/3 -> Switch2/3
  Demux3/1 -> Switch3/1
  Demux3/2 -> Switch3/2
  Demux3/3 -> Switch3/3
  Demux4/1 -> Switch4/1
  Demux4/2 -> Switch4/2
  Demux4/3 -> Switch4/3
  Demux5/1 -> Switch5/1
  Demux5/2 -> Switch5/2
  Demux5/3 -> Switch5/3
  Selector1/1 -> Demux1/1
  Selector5/1 -> Demux5/1
  Selector4/1 -> Demux4/1
  Selector3/1 -> Demux3/1
  Selector2/1 -> Demux2/1
  Selector/1 -> Demux/1
  "q[k],pwm change, q[k-1] ach"/1 -> Selector3/1, Selector4/1, Selector5/1, Selector2/1, Selector1/1, Selector/1

== system Robot_control/Ver 2.0 Haptic Robot Control/Motor Driver System/Orien Processing/Calibrate/Calculate offset values/In time window to calibrate ==
  AND : Logic  IconShape=distinctive  AllPortsSameDT=off  OutDataTypeStr=boolean
  Clock1 : Clock
  Constant2 : Constant  Value=Time_to_wait(2)  VectorParams1D=off  SampleTime=-1
  Constant3 : Constant  Value=Time_to_wait(1)  VectorParams1D=off  SampleTime=-1
  Less Than : RelationalOperator  Operator=<  OutDataTypeStr=boolean  RndMeth=Simplest
  Less Than1 : RelationalOperator  Operator=>  OutDataTypeStr=boolean  RndMeth=Simplest
  Out1 : Outport
  wires:
  Less Than/1 -> AND/1
  Constant3/1 -> Less Than1/2
  Clock1/1 -> Less Than1/1, Less Than/1
  Less Than1/1 -> AND/2
  Constant2/1 -> Less Than/2
  AND/1 -> Out1/1

== system Robot_control/Ver 2.0 Haptic Robot Control/Motor Driver System/Subsystem2/Select pos or orientation mode/If keyboard changes from o->p or p->o then wait 3 sec/Enabled Subsystem ==
  Enable : EnablePort
  Constant : Constant
  MATLAB Function : MATLAB Function  TreatAsAtomicUnit=on
  Terminator : Terminator
  wires:
  Constant/1 -> MATLAB Function/1(u)
  MATLAB Function/1(y) -> Terminator/1

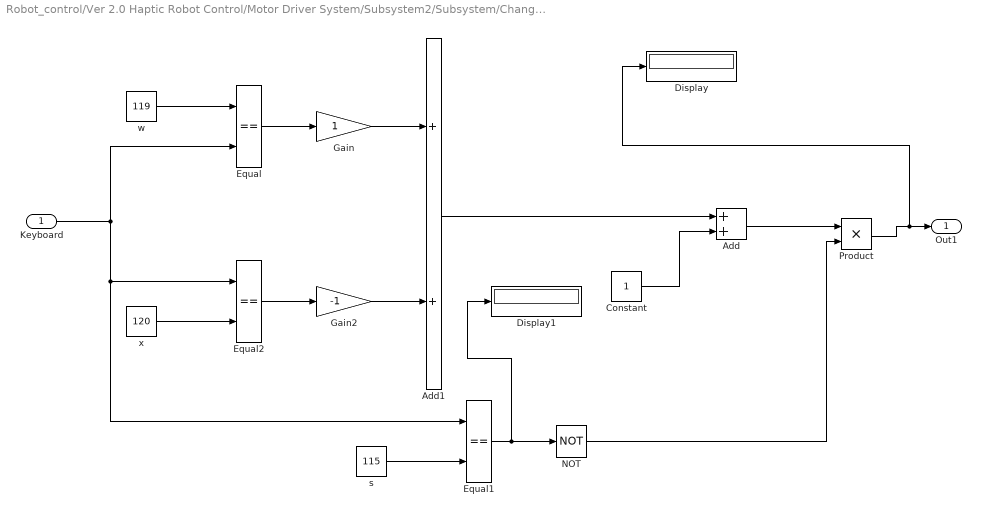
== system Robot_control/Ver 2.0 Haptic Robot Control/Motor Driver System/Subsystem2/Subsystem/Change in Z/w up 1cm s down 1cm ==
  Keyboard : Inport
  Add : Sum
  Add1 : Sum
  Constant : Constant
  Display : Display
  Display1 : Display
  Equal : RelationalOperator  Operator===  OutDataTypeStr=boolean  RndMeth=Simplest
  Equal1 : RelationalOperator  Operator===  OutDataTypeStr=boolean  RndMeth=Simplest
  Equal2 : RelationalOperator  Operator===  OutDataTypeStr=boolean  RndMeth=Simplest
  Gain : Gain
  Gain2 : Gain  Gain=-1
  NOT : Logic  Operator=NOT  IconShape=distinctive  AllPortsSameDT=off  OutDataTypeStr=boolean
  Product : Product
  s : Constant  Value=115
  w : Constant  Value=119
  x : Constant  Value=120
  Out1 : Outport
  wires:
  w/1 -> Equal/1
  Equal/1 -> Gain/1
  Gain/1 -> Add1/1
  Constant/1 -> Add/2
  Add/1 -> Product/1
  Equal2/1 -> Gain2/1
  x/1 -> Equal2/2
  Gain2/1 -> Add1/2
  Add1/1 -> Add/1
  Keyboard/1 -> Equal/2, Equal1/1, Equal2/1
  s/1 -> Equal1/2
  Equal1/1 -> Display1/1, NOT/1
  NOT/1 -> Product/2
  Product/1 -> Display/1, Out1/1

== system Robot_control/Ver 2.0 Haptic Robot Control/Motor Driver System/Subsystem2/Subsystem/Hysteresis/Subsystem ==
  angular pos after Cal : Inport
  Dot Product : DotProduct  InputSameDT=on  OutDataTypeStr=Inherit: Inherit via internal rule
  Sqrt : Sqrt  SaturateOnIntegerOverflow=on
  Transpose : Math  Operator=transpose  SaturateOnIntegerOverflow=on
  angular pos magnitude : Outport
  wires:
  Dot Product/1 -> Sqrt/1
  Transpose/1 -> Dot Product/2
  Sqrt/1 -> angular pos magnitude/1
  angular pos after Cal/1 -> Dot Product/1, Transpose/1

== matlab function Robot_control/Ver 2.0 Haptic Robot Control/Tooltip System/Subsystem1/MATLAB Function1 ==
  data: y output size=[1 2]; my_string input string [0..100]
function y  = str_com2_array(my_string)
y = [0 0];
%coder.varsize('my_string',[1 100]);
char_array = convertStringsToChars(my_string);
j=1;
i=1;
count = 0;
markNeg = 0;
while i <= length(char_array)
    if(char_array(i) == '-')
        markNeg = 1;
    end
    
    if(char_array(i)== ',')
        if(markNeg == 1)
            if(count == 2)
                y(j)=real(-1*str2double(char_array(i-1)));
            elseif(count == 3)
                y(j)=real(-1*((str2double(char_array(i-2))*10) + (str2double(char_array(i-1)))));
            elseif(count == 4)
                y(j)=real(-1*((str2double(char_array(i-3))*100) + (str2double(char_array(i-2))*10) + (str2double(char_array(i-1)))));
            elseif(count == 5)
                y(j)=real(-1*((str2double(char_array(i-4))*1000) + (str2double(char_array(i-3))*100) + (str2double(char_array(i-2))*10) + (str2double(char_array(i-1)))));
            elseif(count == 6)
                y(j)=real(-1*((str2double(char_array(i-5))*10000) + (str2double(char_array(i-4))*1000) + (str2double(char_array(i-3))*100) + (str2double(char_array(i-2))*10) + (str2double(char_array(i-1)))));
            end
        else
            if(count == 1)
                y(j)=real(str2double(char_array(i-1)));
            elseif(count == 2)
                y(j)=real((str2double(char_array(i-2))*10) + (str2double(char_array(i-1))));
            elseif(count == 3)
                y(j)=real((str2double(char_array(i-3))*100) + (str2double(char_array(i-2))*10) + (str2double(char_array(i-1))));
            elseif(count == 4)
                y(j)=real((str2double(char_array(i-4))*1000) + (str2double(char_array(i-3))*100) +  + (str2double(char_array(i-2))*10) + (str2double(char_array(i-1))));
            elseif(count == 5)
                y(j)=real((str2double(char_array(i-5))*10000) + (str2double(char_array(i-4))*1000) + (str2double(char_array(i-3))*100) + (str2double(char_array(i-2))*10) + (str2double(char_array(i-1))));
            end
        end
        j=j+1;
        count = 0;
        markNeg = 0;
    else
        count = count + 1;
        if(i == length(char_array))
            if(markNeg == 1)
                if(count == 2)
                    y(j)=real(-1*str2double(char_array(i)));
                elseif(count == 3)
                    y(j)=real(-1*((str2double(char_array(i-1))*10) + (str2double(char_array(i)))));
                elseif(count == 4)
                    y(j)=real(-1*((str2double(char_array(i-2))*100) + (str2double(char_array(i-1))*10) + (str2double(char_array(i)))));
                elseif(count == 5)
                    y(j)=real(-1*((str2double(char_array(i-3))*1000) + (str2double(char_array(i-2))*100) +  + (str2double(char_array(i-1))*10) + (str2double(char_array(i)))));
                elseif(count == 6)
                    y(j)=real(-1*((str2double(char_array(i-4))*10000) + (str2double(char_array(i-3))*1000) + (str2double(char_array(i-2))*100) + (str2double(char_array(i-1))*10) + (str2double(char_array(i)))));
                end
            else
                if(count == 1)
                    y(j)=real(str2double(char_array(i)));
                elseif(count == 2)
                    y(j)=real((str2double(char_array(i-1))*10) + (str2double(char_array(i))));
                elseif(count == 3)
                    y(j)=real((str2double(char_array(i-2))*100) + (str2double(char_array(i-1))*10) + (str2double(char_array(i))));
                elseif(count == 4)
                    y(j)=real((str2double(char_array(i-3))*1000) + (str2double(char_array(i-2))*100) +  + (str2double(char_array(i-1))*10) + (str2double(char_array(i))));
                elseif(count == 5)
                    y(j)=real((str2double(char_array(i-4))*10000) + (str2double(char_array(i-3))*1000) + (str2double(char_array(i-2))*100) + (str2double(char_array(i-1))*10) + (str2double(char_array(i))));
                end
            end
        end
    end
    i = i+1;
end
end

== matlab function Robot_control/Ver 2.0 Haptic Robot Control/Motor Driver System/Subsystem2/Select pos or orientation mode/If keyboard changes from o->p or p->o then wait 3 sec/Enabled Subsystem/MATLAB Function ==
  data: u input; y output
function y = fcn(u)
pause(3)
y = u;

== matlab function Robot_control/Ver 2.0 Haptic Robot Control/Motor Driver System/ESP32 Right glove read/Triggered Subsystem/MATLAB Function1 ==
  data: y output size=[1 9]; my_string input string [0..100]
function y  = str_com2_array(my_string)
y = [0 0 0 0 0 0 0 0 0];
%coder.varsize('my_string',[1 100]);
char_array = convertStringsToChars(my_string);
j=1;
i=1;
count = 0;
markNeg = 0;
while i <= length(char_array)
    if(char_array(i) == '-')
        markNeg = 1;
    end
    
    if(char_array(i)== ',')
        if(markNeg == 1)
            if(count == 2)
                y(j)=real(-1*str2double(char_array(i-1)));
            elseif(count == 3)
                y(j)=real(-1*((str2double(char_array(i-2))*10) + (str2double(char_array(i-1)))));
            elseif(count == 4)
                y(j)=real(-1*((str2double(char_array(i-3))*100) + (str2double(char_array(i-2))*10) + (str2double(char_array(i-1)))));
            elseif(count == 5)
                y(j)=real(-1*((str2double(char_array(i-4))*1000) + (str2double(char_array(i-3))*100) + (str2double(char_array(i-2))*10) + (str2double(char_array(i-1)))));
            elseif(count == 6)
                y(j)=real(-1*((str2double(char_array(i-5))*10000) + (str2double(char_array(i-4))*1000) + (str2double(char_array(i-3))*100) + (str2double(char_array(i-2))*10) + (str2double(char_array(i-1)))));
            end
        else
            if(count == 1)
                y(j)=real(str2double(char_array(i-1)));
            elseif(count == 2)
                y(j)=real((str2double(char_array(i-2))*10) + (str2double(char_array(i-1))));
            elseif(count == 3)
                y(j)=real((str2double(char_array(i-3))*100) + (str2double(char_array(i-2))*10) + (str2double(char_array(i-1))));
            elseif(count == 4)
                y(j)=real((str2double(char_array(i-4))*1000) + (str2double(char_array(i-3))*100) +  + (str2double(char_array(i-2))*10) + (str2double(char_array(i-1))));
            elseif(count == 5)
                y(j)=real((str2double(char_array(i-5))*10000) + (str2double(char_array(i-4))*1000) + (str2double(char_array(i-3))*100) + (str2double(char_array(i-2))*10) + (str2double(char_array(i-1))));
            end
        end
        j=j+1;
        count = 0;
        markNeg = 0;
    else
        count = count + 1;
        if(i == length(char_array))
            if(markNeg == 1)
                if(count == 2)
                    y(j)=real(-1*str2double(char_array(i)));
                elseif(count == 3)
                    y(j)=real(-1*((str2double(char_array(i-1))*10) + (str2double(char_array(i)))));
                elseif(count == 4)
                    y(j)=real(-1*((str2double(char_array(i-2))*100) + (str2double(char_array(i-1))*10) + (str2double(char_array(i)))));
                elseif(count == 5)
                    y(j)=real(-1*((str2double(char_array(i-3))*1000) + (str2double(char_array(i-2))*100) +  + (str2double(char_array(i-1))*10) + (str2double(char_array(i)))));
                elseif(count == 6)
                    y(j)=real(-1*((str2double(char_array(i-4))*10000) + (str2double(char_array(i-3))*1000) + (str2double(char_array(i-2))*100) + (str2double(char_array(i-1))*10) + (str2double(char_array(i)))));
                end
            else
                if(count == 1)
                    y(j)=real(str2double(char_array(i)));
                elseif(count == 2)
                    y(j)=real((str2double(char_array(i-1))*10) + (str2double(char_array(i))));
                elseif(count == 3)
                    y(j)=real((str2double(char_array(i-2))*100) + (str2double(char_array(i-1))*10) + (str2double(char_array(i))));
                elseif(count == 4)
                    y(j)=real((str2double(char_array(i-3))*1000) + (str2double(char_array(i-2))*100) +  + (str2double(char_array(i-1))*10) + (str2double(char_array(i))));
                elseif(count == 5)
                    y(j)=real((str2double(char_array(i-4))*10000) + (str2double(char_array(i-3))*1000) + (str2double(char_array(i-2))*100) + (str2double(char_array(i-1))*10) + (str2double(char_array(i))));
                end
            end
        end
    end
    i = i+1;
end
end

== matlab function Robot_control/Ver 2.0 Haptic Robot Control/Motor Driver System/Orien Processing/Kalman and AHRS/Kalman Filter for Pitch ==
  data: dt input; pitch output; Q_angle input; Q_bias input; R input; newAngle input; newRate input; P_temp output; K output; bias output; y output; rate output
function [pitch, P_temp, K, bias, y, rate]  = kalFilterPitch(dt, Q_angle, Q_bias, R, newAngle, newRate)

persistent angle;
persistent P;


%Process Noise Convariance Matrix
Q = [Q_angle 0; 0 Q_bias] * dt;
F = [1  -dt; 0 1];
H = [1 0];
bias = 0.0;

rate = newRate - bias;

if isempty(angle); angle = 0;
    
else angle = angle + (dt * rate);
end 

pitch = angle;

if isempty(P); P = [0, 0; 0, 0];
else P = F*P*F' + Q;
end 
P_temp = P;

S = H*P*H' + R;
K = (P_temp * H')/S;
y = newAngle - pitch; 
pitch = pitch + K(1) * y;
bias = pitch + K(2) * y;
angle = pitch;

I = [1 0; 0 1];
P_temp = (I - K*H)*P_temp;
P = P_temp;

return 


end

== matlab function Robot_control/Ver 2.0 Haptic Robot Control/Motor Driver System/Orien Processing/Kalman and AHRS/Kalman Filter for Roll ==
  data: dt input; roll output; Q_angle input; Q_bias input; R input; newAngle input; newRate input; P_temp output; K output; bias output; y output; rate output
function [roll, P_temp, K, bias, y, rate]  = kalFilterRoll(dt, Q_angle, Q_bias, R, newAngle, newRate)

persistent angle;
persistent P;


%Process Noise Convariance Matrix
Q = [Q_angle 0; 0 Q_bias] * dt;
F = [1  -dt; 0 1];
H = [1 0];
bias = 0.0;

rate = newRate - bias;

if isempty(angle); angle = 0;
    
else angle = angle + (dt * rate);
end 

roll = angle;

if isempty(P); P = [0, 0; 0, 0];
else P = F*P*F' + Q;
end 
P_temp = P;

S = H*P*H' + R;
K = (P_temp * H')/S;
y = newAngle - roll; 
roll = roll + K(1) * y;
bias = roll + K(2) * y;
angle = roll;

I = [1 0; 0 1];
P_temp = (I - K*H)*P_temp;
P = P_temp;

return 


end
